simulink model "matprob7"  (R2020a)
settings: Solver=VariableStepAuto  StartTime=0.0  StopTime=10.0  RelTol=1e-3
libraries: simulink x1
settings Model: Creator=deepa  LastModifiedBy=deepa

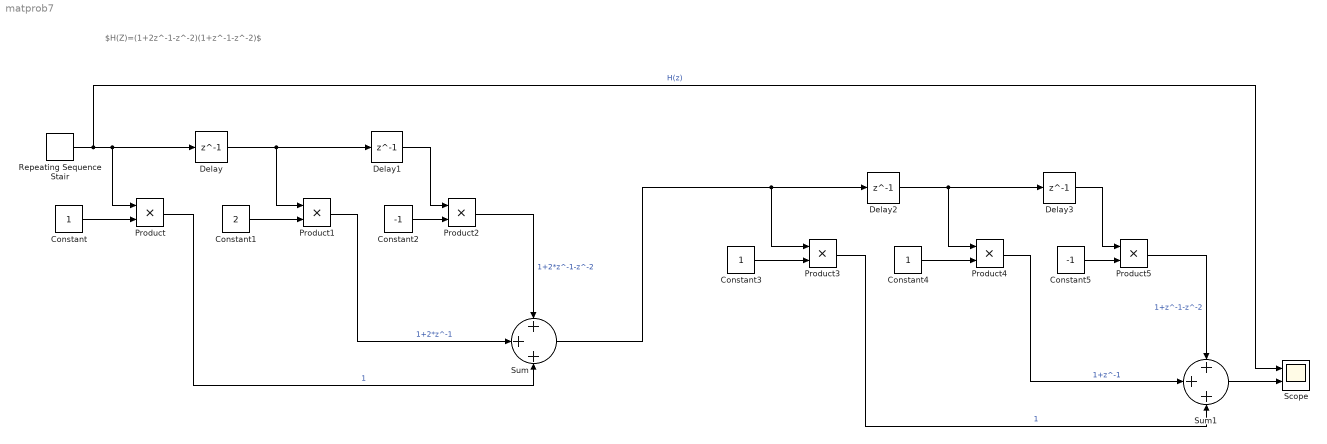
== system matprob7 ==
  note: $H(Z)=(1+2z^-1-z^-2)(1+z^-1-z^-2)$
  Constant : Constant
  Constant1 : Constant  Value=2
  Constant2 : Constant  Value=-1
  Constant3 : Constant
  Constant4 : Constant
  Constant5 : Constant  Value=-1
  Delay{,1..3} (4 alike) : Delay  DelayLength=1
  Product{,1..5} (6 alike) : Product
  Repeating Sequence Stair : simulink/Sources/Repeating Sequence Stair  OutValues=[3 1 4 2 1].'  tsamp=-1  OutMin=[]  OutMax=[]  OutDataTypeStr=double  OutputDataTypeScalingMode=double  OutDataType=fixdt(0,8)  ConRadixGroup=Best Precision: Vector-wise  OutScaling=2^-12
  Scope : Scope  NumInputPorts=2
  Sum : Sum  Inputs=+++
  Sum1 : Sum  Inputs=+++
  wires:
  Repeating Sequence Stair/1 -> Scope/1, Product/1, Delay/1  "H(z)"
  Delay/1 -> Product1/1, Delay1/1
  Constant/1 -> Product/2
  Constant1/1 -> Product1/2
  Constant2/1 -> Product2/2
  Delay1/1 -> Product2/1
  Product2/1 -> Sum/1  "1+2*z^-1-z^-2"
  Product1/1 -> Sum/2  "1+2*z^-1"
  Product/1 -> Sum/3  "1"
  Product4/1 -> Sum1/2  "1+z^-1"
  Delay3/1 -> Product5/1
  Constant5/1 -> Product5/2
  Product5/1 -> Sum1/1  "1+z^-1-z^-2"
  Delay2/1 -> Product4/1, Delay3/1
  Constant3/1 -> Product3/2
  Product3/1 -> Sum1/3  "1"
  Constant4/1 -> Product4/2
  Sum/1 -> Product3/1, Delay2/1
  Sum1/1 -> Scope/2
